simulink model "ball_simulink_restored_from_autosave"  (R2019b)
settings: Solver=VariableStepAuto  StartTime=0.0  StopTime=10  RelTol=1e-3
libraries: simulink x1
settings Model: Creator=Δημήτρης  LastModifiedBy=Εμμανουήλ
settings SolverCC: ShapePreserveControl=EnableAll

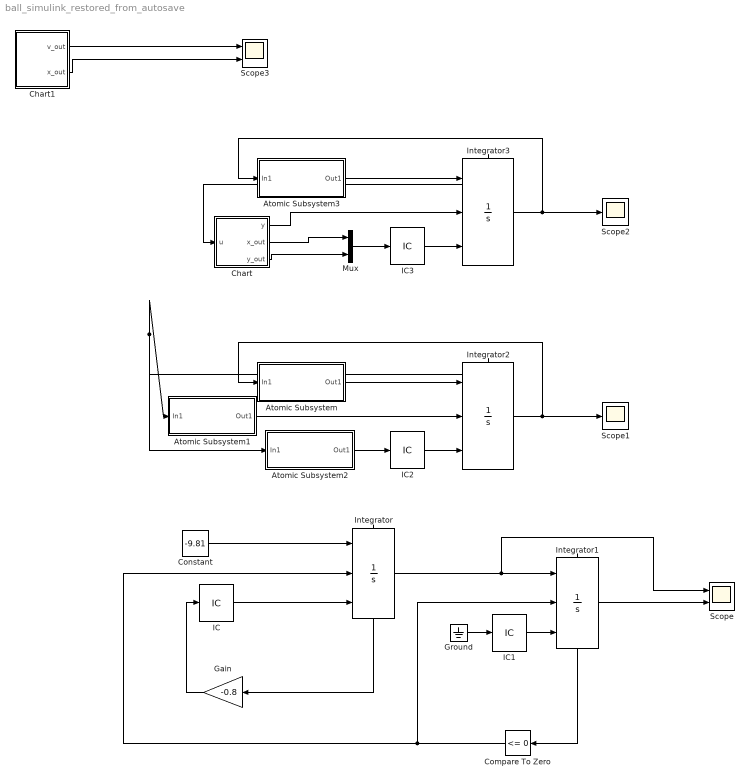
== system ball_simulink_restored_from_autosave ==
  Atomic Subsystem : Subsystem  TreatAsAtomicUnit=on
  Atomic Subsystem1 : Subsystem  TreatAsAtomicUnit=on
  Atomic Subsystem2 : Subsystem  TreatAsAtomicUnit=on
  Atomic Subsystem3 : Subsystem  TreatAsAtomicUnit=on
  Chart : Stateflow chart  BlockKeywords=__PRM__SERIALIZED__DATA__:Stateflow Chart,Stateflow Diagram  TreatAsAtomicUnit=on
  Chart1 : Stateflow chart  BlockKeywords=__PRM__SERIALIZED__DATA__:Stateflow Chart,Stateflow Diagram  TreatAsAtomicUnit=on
  Compare To Zero : simulink/Logic and Bit Operations/Compare To Zero  relop=<=  OutDataTypeStr=boolean
  Constant : Constant  Value=-9.81
  Gain : Gain  Gain=-0.8
  Ground : Ground
  IC : InitialCondition  Value=15
  IC1 : InitialCondition  Value=10
  IC2 : InitialCondition  Value=[10;15]
  IC3 : InitialCondition  Value=[10;15]
  Integrator : Integrator  ExternalReset=rising  InitialConditionSource=external  ShowStatePort=on
  Integrator1 : Integrator  ExternalReset=rising  InitialConditionSource=external  LimitOutput=on  ShowStatePort=on  IgnoreLimit=on
  Integrator2 : Integrator  ExternalReset=rising  InitialConditionSource=external  ShowStatePort=on  IgnoreLimit=on
  Integrator3 : Integrator  ExternalReset=rising  InitialConditionSource=external  ShowStatePort=on  IgnoreLimit=on
  Mux : Mux  Inputs=2
  Scope : Scope  NumInputPorts=2
  Scope1 : Scope
  Scope2 : Scope
  Scope3 : Scope  NumInputPorts=2
  wires:
  IC/1 -> Integrator/3
  Gain/1 -> IC/1
  Constant/1 -> Integrator/1
  Integrator/State -> Gain/1
  Integrator/1 -> Scope/1, Integrator1/1
  Integrator1/State -> Compare To Zero/1
  Compare To Zero/1 -> Integrator1/2, Integrator/2
  IC1/1 -> Integrator1/3
  Ground/1 -> IC1/1
  Integrator1/1 -> Scope/2
  Atomic Subsystem/1(Out1) -> Integrator2/1
  Atomic Subsystem1/1(Out1) -> Integrator2/2
  IC2/1 -> Integrator2/3
  Atomic Subsystem2/1(Out1) -> IC2/1
  Integrator2/1 -> Scope1/1, Atomic Subsystem/1(In1)
  Integrator2/State -> Atomic Subsystem1/1(In1), Atomic Subsystem2/1(In1)
  Integrator3/1 -> Atomic Subsystem3/1(In1), Scope2/1
  Chart/2(x_out) -> Mux/1
  Mux/1 -> IC3/1
  Atomic Subsystem3/1(Out1) -> Integrator3/1
  Integrator3/State -> Chart/1(u)
  Chart/3(y_out) -> Mux/2
  Chart/1(y) -> Integrator3/2
  IC3/1 -> Integrator3/3
  Chart1/1(v_out) -> Scope3/1
  Chart1/2(x_out) -> Scope3/2

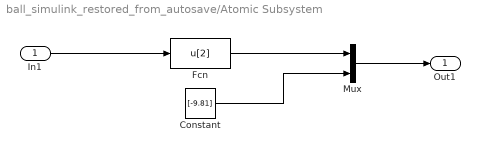
== system ball_simulink_restored_from_autosave/Atomic Subsystem ==
  In1 : Inport
  Constant : Constant  Value=[-9.81]
  Fcn : Fcn  Expr=u[2]
  Mux : Mux  Inputs=2
  Out1 : Outport
  wires:
  Mux/1 -> Out1/1
  Fcn/1 -> Mux/1
  In1/1 -> Fcn/1
  Constant/1 -> Mux/2

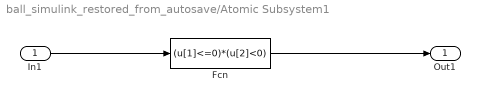
== system ball_simulink_restored_from_autosave/Atomic Subsystem1 ==
  In1 : Inport
  Fcn : Fcn  Expr=(u[1]<=0)*(u[2]<0)
  Out1 : Outport
  wires:
  In1/1 -> Fcn/1
  Fcn/1 -> Out1/1

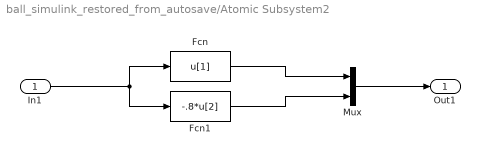
== system ball_simulink_restored_from_autosave/Atomic Subsystem2 ==
  In1 : Inport
  Fcn : Fcn  Expr=u[1]
  Fcn1 : Fcn  Expr=-.8*u[2]
  Mux : Mux  Inputs=2
  Out1 : Outport
  wires:
  Mux/1 -> Out1/1
  Fcn/1 -> Mux/1
  In1/1 -> Fcn1/1, Fcn/1
  Fcn1/1 -> Mux/2

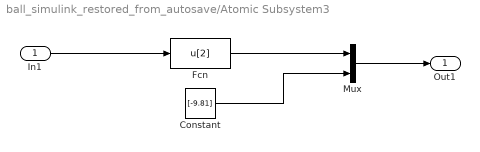
== system ball_simulink_restored_from_autosave/Atomic Subsystem3 ==
  In1 : Inport
  Constant : Constant  Value=[-9.81]
  Fcn : Fcn  Expr=u[2]
  Mux : Mux  Inputs=2
  Out1 : Outport
  wires:
  Constant/1 -> Mux/2
  In1/1 -> Fcn/1
  Fcn/1 -> Mux/1
  Mux/1 -> Out1/1

== stateflow chart ball_simulink_restored_from_autosave/Chart ==
  state on
    entry:y=0;
  state off
    entry:y=1;
    x_out=u(1);
    y_out=-0.8*u(2);
  (default) -> on
  on -> off : [u(1)<=0&&u(2)<0]
  off -> on
  data: y output; x_out output; y_out output; u input

== stateflow chart ball_simulink_restored_from_autosave/Chart1 ==
  settings: updateMethod=CONTINUOUS  executeAtInitialization=1  initializeOutput=1
  state BALL
    du:
    x_dot = v;
    v_dot = -9.81;
    %outputs
    x_out = x;
    v_out = v;
  (default) -> BALL : {
      | x = 10;
      | v = 15;
      | }
  BALL -> BALL : [x<=0&&v<0]
      | {x = 0;
      | v = -0.8.*v;}
  data: v_out output double; x local double; v local double; x_out output double
  data x settings: updateMethod=SF_CONTINUOUS_TIME_DATA
  data v settings: updateMethod=SF_CONTINUOUS_TIME_DATA
